simulink model "sampleModel2432_pp_1_2"  (R2018a)
settings: Solver=VariableStepAuto  StartTime=0.0  StopTime=10.0  RelTol=1e-3
undefined symbols (not defined in the file or in its folder): DiscIntNeverNeededParam, sigbuilder_block
libraries: simulink x302
(part 6 of 7)

== system sampleModel2432_pp_1_2/cfblk225/cfblk17 ==
  cfblk1 : Inport
  Action Port : ActionPort
  cfblk{10,15..17} (4 alike) : Delay
  cfblk14 : simulink/Discrete/Transfer Fcn Lead or Lag  PoleZ=0.95  ZeroZ=0.75  ICPrevOutput=0.0  ICPrevInput=0.0  DoSatur=off
      settings: SourceProductName=Simulink  SourceProductBaseCode=SL
  cfblk3 : DiscreteFilter
  cfblk4 : simulink/Continuous/PID Controller (2DOF)  Controller=PID  TimeDomain=Discrete-time  SampleTime=-1  IntegratorMethod=Forward Euler  FilterMethod=Forward Euler  Form=Parallel  UseFilter=on  ControllerParametersSource=internal  P=1  I=1  D=0  N=100  b=1  c=1  InitialConditionSource=internal  InitialConditionForIntegrator=0  InitialConditionForFilter=0  ExternalReset=none  LimitOutput=off  UpperSaturationLimit=inf  LowerSaturationLimit=-inf  LinearizeAsGain=off  AntiWindupMode=none  Kb=1  TrackingMode=off  Kt=1  PParamMin=[]  PParamMax=[]  IParamMin=[]  IParamMax=[]  DParamMin=[]  DParamMax=[]  NParamMin=[]  NParamMax=[]  bParamMin=[]  bParamMax=[]  cParamMin=[]  cParamMax=[]  KbParamMin=[]  KbParamMax=[]  KtParamMin=[]  KtParamMax=[]  POutMin=[]  POutMax=[]  IOutMin=[]  IOutMax=[]  DOutMin=[]  DOutMax=[]  NOutMin=[]  NOutMax=[]  bOutMin=[]  bOutMax=[]  cOutMin=[]  cOutMax=[]  KbOutMin=[]  KbOutMax=[]  KtOutMin=[]  KtOutMax=[]  IntegratorOutMin=[]  IntegratorOutMax=[]  FilterOutMin=[]  FilterOutMax=[]  SumOutMin=[]  SumOutMax=[]  Sum1OutMin=[]  Sum1OutMax=[]  Sum2OutMin=[]  Sum2OutMax=[]  Sum3OutMin=[]  Sum3OutMax=[]  SumI1OutMin=[]  SumI1OutMax=[]  SumI2OutMin=[]  SumI2OutMax=[]  SumI3OutMin=[]  SumI3OutMax=[]  SumDOutMin=[]  SumDOutMax=[]  SaturationOutMin=[]  SaturationOutMax=[]  IntegratorContinuousStateAttributes=''  IntegratorStateMustResolveToSignalObject=off  IntegratorRTWStateStorageClass=Auto  FilterContinuousStateAttributes=''  FilterStateMustResolveToSignalObject=off  FilterRTWStateStorageClass=Auto  DifferentiatorICPrevScaledInput=0  DifferentiatorOutMin=[]  DifferentiatorOutMax=[]  FilterDiffOutCoefMin=[]  FilterDiffOutCoefMax=[]  SumDenOutMin=[]  SumDenOutMax=[]  SumNumOutMin=[]  SumNumOutMax=[]  ReciprocalOutMin=[]  ReciprocalOutMax=[]  DivideOutMin=[]  DivideOutMax=[]  TunerSelectOption=Transfer Function Based (PID Tuner App)
  cfblk6 : DiscreteStateSpace  SampleTime=-1
  cfblk7 : DiscreteTransferFcn
  cfblk8 : Delay  DelayLengthSource=Input port
      settings: InputPortMap=u0,p1
  cyemi_{709..726} (18 alike) : DataTypeConversion  OutDataTypeStr=double
  cfblk2 : Outport
  wires:
  cfblk1/1 -> cyemi_709/1, cyemi_719/1
  cfblk6/1 -> cfblk2/1
  cyemi_709/1 -> cfblk10/1
  cfblk8/1 -> cyemi_710/1
  cyemi_713/1 -> cfblk14/1
  cyemi_714/1 -> cfblk15/1
  cfblk7/1 -> cyemi_714/1
  cyemi_715/1 -> cfblk16/1
  cyemi_716/1 -> cfblk17/1
  cyemi_717/1 -> cfblk3/1
  cfblk4/1 -> cyemi_717/1
  cyemi_718/1 -> cfblk4/1
  cfblk15/1 -> cyemi_718/1
  cyemi_719/1 -> cfblk4/2
  cyemi_721/1 -> cfblk6/1
  cfblk10/1 -> cyemi_721/1
  cyemi_722/1 -> cfblk7/1
  cfblk14/1 -> cyemi_722/1
  cyemi_723/1 -> cfblk8/1
  cfblk3/1 -> cyemi_723/1
  cyemi_724/1 -> cfblk8/2
  cfblk17/1 -> cyemi_724/1
  cfblk16/1 -> cyemi_725/1
  cyemi_725/1 -> cyemi_720/1
  cyemi_711/1 -> cyemi_715/1
  cyemi_712/1 -> cyemi_726/1, cyemi_713/1
  cyemi_710/1 -> cyemi_716/1, cyemi_712/1
  cyemi_720/1 -> cyemi_711/1

== system sampleModel2432_pp_1_2/cfblk227/cfblk13 ==
  cfblk1 : Inport
  cfblk13 : Inport  Port=2
  cfblk14 : Inport  Port=3
  Action Port : ActionPort  ActionType=then
  cfblk10 : Delay  DelayLengthSource=Input port
      settings: InputPortMap=u0,p1
  cfblk11 : simulink/Discrete/Difference  ICPrevInput=0.0  OutMin=[]  OutMax=[]  OutDataTypeStr=Inherit: Inherit via back propagation  OutDataType=fixdt(1, 16)  OutScaling=2^-10  DoSatur=off
  cfblk16 : Delay
  cfblk3 : simulink/Discrete/Difference  ICPrevInput=0.0  OutMin=[]  OutMax=[]  OutDataTypeStr=Inherit: Inherit via back propagation  OutDataType=fixdt(1, 16)  OutScaling=2^-10  DoSatur=off
  cfblk5 : UnitDelay  SampleTime=-1
  cfblk6 : Delay
  cfblk7 : Delay  ShowEnablePort=on
      settings: InputPortMap=u0,e6
  cfblk9 : simulink/Discrete/Transfer Fcn Real Zero  ZeroZ=0.75  ICPrevInput=0.0  DoSatur=off
      settings: SourceProductName=Simulink  SourceProductBaseCode=SL
  cyemi_{761..774} (14 alike) : DataTypeConversion  OutDataTypeStr=double
  cfblk2 : Outport
  cfblk15 : Outport  Port=2
  wires:
  cfblk3/1 -> cfblk2/1
  cfblk13/1 -> cyemi_763/1, cyemi_774/1
  cyemi_761/1 -> cfblk10/1
  cfblk14/1 -> cyemi_761/1
  cyemi_762/1 -> cfblk10/2
  cfblk5/1 -> cyemi_762/1
  cyemi_763/1 -> cfblk11/1
  cfblk11/1 -> cyemi_764/1
  cfblk6/1 -> cyemi_765/1
  cyemi_766/1 -> cfblk16/1
  cyemi_767/1 -> cfblk3/1
  cfblk9/1 -> cyemi_768/1
  cyemi_769/1 -> cfblk5/1
  cyemi_770/1 -> cfblk6/1
  cfblk7/1 -> cyemi_770/1
  cyemi_771/1 -> cfblk7/1
  cfblk10/1 -> cyemi_771/1
  cyemi_772/1 -> cfblk7/2
  cfblk16/1 -> cyemi_772/1
  cfblk1/1 -> cyemi_773/1
  cyemi_774/1 -> cfblk9/1
  cyemi_768/1 -> cyemi_769/1, cfblk15/1
  cyemi_764/1 -> cyemi_766/1
  cyemi_773/1 -> cyemi_767/1

== system sampleModel2432_pp_1_2/cfblk227/cfblk14 ==
  cfblk1 : Inport
  cfblk6 : Inport  Port=2
  Action Port : ActionPort  ActionType=else
  cfblk3 : simulink/Discrete/Tapped Delay  vinit=0.0  samptime=-1  NumDelays=1  DelayOrder=Oldest  includeCurrent=off
  cfblk4 : simulink/Discrete/Difference  ICPrevInput=0.0  OutMin=[]  OutMax=[]  OutDataTypeStr=Inherit: Inherit via back propagation  OutDataType=fixdt(1, 16)  OutScaling=2^-10  DoSatur=off
  cyemi_777 : DataTypeConversion  OutDataTypeStr=double
  cyemi_778 : DataTypeConversion  OutDataTypeStr=double
  cyemi_779 : DataTypeConversion  OutDataTypeStr=double
  cfblk2 : Outport
  cfblk7 : Outport  Port=2
  wires:
  cfblk3/1 -> cfblk2/1
  cfblk4/1 -> cfblk7/1
  cyemi_777/1 -> cfblk3/1
  cfblk6/1 -> cyemi_777/1
  cyemi_778/1 -> cfblk4/1
  cfblk1/1 -> cyemi_779/1
  cyemi_779/1 -> cyemi_778/1

== system sampleModel2432_pp_1_2/cfblk230/cfblk10 ==
  cfblk1 : Inport
  Action Port : ActionPort  ActionType=then
  cfblk10 : UnitDelay  SampleTime=-1
  cfblk13 : Delay
  cfblk14 : Delay
  cfblk3 : simulink/Continuous/PID Controller (2DOF)  Controller=PID  TimeDomain=Discrete-time  SampleTime=-1  IntegratorMethod=Forward Euler  FilterMethod=Forward Euler  Form=Parallel  UseFilter=on  ControllerParametersSource=internal  P=1  I=1  D=0  N=100  b=1  c=1  InitialConditionSource=internal  InitialConditionForIntegrator=0  InitialConditionForFilter=0  ExternalReset=none  LimitOutput=off  UpperSaturationLimit=inf  LowerSaturationLimit=-inf  LinearizeAsGain=off  AntiWindupMode=none  Kb=1  TrackingMode=off  Kt=1  PParamMin=[]  PParamMax=[]  IParamMin=[]  IParamMax=[]  DParamMin=[]  DParamMax=[]  NParamMin=[]  NParamMax=[]  bParamMin=[]  bParamMax=[]  cParamMin=[]  cParamMax=[]  KbParamMin=[]  KbParamMax=[]  KtParamMin=[]  KtParamMax=[]  POutMin=[]  POutMax=[]  IOutMin=[]  IOutMax=[]  DOutMin=[]  DOutMax=[]  NOutMin=[]  NOutMax=[]  bOutMin=[]  bOutMax=[]  cOutMin=[]  cOutMax=[]  KbOutMin=[]  KbOutMax=[]  KtOutMin=[]  KtOutMax=[]  IntegratorOutMin=[]  IntegratorOutMax=[]  FilterOutMin=[]  FilterOutMax=[]  SumOutMin=[]  SumOutMax=[]  Sum1OutMin=[]  Sum1OutMax=[]  Sum2OutMin=[]  Sum2OutMax=[]  Sum3OutMin=[]  Sum3OutMax=[]  SumI1OutMin=[]  SumI1OutMax=[]  SumI2OutMin=[]  SumI2OutMax=[]  SumI3OutMin=[]  SumI3OutMax=[]  SumDOutMin=[]  SumDOutMax=[]  SaturationOutMin=[]  SaturationOutMax=[]  IntegratorContinuousStateAttributes=''  IntegratorStateMustResolveToSignalObject=off  IntegratorRTWStateStorageClass=Auto  FilterContinuousStateAttributes=''  FilterStateMustResolveToSignalObject=off  FilterRTWStateStorageClass=Auto  DifferentiatorICPrevScaledInput=0  DifferentiatorOutMin=[]  DifferentiatorOutMax=[]  FilterDiffOutCoefMin=[]  FilterDiffOutCoefMax=[]  SumDenOutMin=[]  SumDenOutMax=[]  SumNumOutMin=[]  SumNumOutMax=[]  ReciprocalOutMin=[]  ReciprocalOutMax=[]  DivideOutMin=[]  DivideOutMax=[]  TunerSelectOption=Transfer Function Based (PID Tuner App)
  cfblk5 : DiscreteFir
  cfblk6 : UnitDelay  SampleTime=-1
  cfblk8 : simulink/Continuous/PID Controller  Controller=PID  TimeDomain=Discrete-time  SampleTime=-1  IntegratorMethod=Forward Euler  FilterMethod=Forward Euler  Form=Parallel  UseFilter=on  ControllerParametersSource=internal  P=1  I=1  D=0  N=100  InitialConditionSource=internal  InitialConditionForIntegrator=0  InitialConditionForFilter=0  ExternalReset=none  LimitOutput=off  UpperSaturationLimit=inf  LowerSaturationLimit=-inf  LinearizeAsGain=off  AntiWindupMode=none  Kb=1  TrackingMode=off  Kt=1  PParamMin=[]  PParamMax=[]  IParamMin=[]  IParamMax=[]  DParamMin=[]  DParamMax=[]  NParamMin=[]  NParamMax=[]  KbParamMin=[]  KbParamMax=[]  KtParamMin=[]  KtParamMax=[]  POutMin=[]  POutMax=[]  IOutMin=[]  IOutMax=[]  DOutMin=[]  DOutMax=[]  NOutMin=[]  NOutMax=[]  KbOutMin=[]  KbOutMax=[]  KtOutMin=[]  KtOutMax=[]  IntegratorOutMin=[]  IntegratorOutMax=[]  FilterOutMin=[]  FilterOutMax=[]  SumOutMin=[]  SumOutMax=[]  SumI1OutMin=[]  SumI1OutMax=[]  SumI2OutMin=[]  SumI2OutMax=[]  SumI3OutMin=[]  SumI3OutMax=[]  SumDOutMin=[]  SumDOutMax=[]  SaturationOutMin=[]  SaturationOutMax=[]  IntegratorContinuousStateAttributes=''  IntegratorStateMustResolveToSignalObject=off  IntegratorRTWStateStorageClass=Auto  FilterContinuousStateAttributes=''  FilterStateMustResolveToSignalObject=off  FilterRTWStateStorageClass=Auto  DifferentiatorICPrevScaledInput=0  DifferentiatorOutMin=[]  DifferentiatorOutMax=[]  FilterDiffOutCoefMin=[]  FilterDiffOutCoefMax=[]  SumDenOutMin=[]  SumDenOutMax=[]  SumNumOutMin=[]  SumNumOutMax=[]  ReciprocalOutMin=[]  ReciprocalOutMax=[]  DivideOutMin=[]  DivideOutMax=[]  TunerSelectOption=Transfer Function Based (PID Tuner App)
  cyemi_{816..826} (11 alike) : DataTypeConversion  OutDataTypeStr=double
  cfblk2 : Outport
  cfblk11 : Outport  Port=2
  cfblk12 : Outport  Port=3
  wires:
  cfblk10/1 -> cfblk12/1, cyemi_821/1
  cfblk6/1 -> cyemi_817/1, cyemi_822/1
  cfblk8/1 -> cfblk2/1
  cfblk5/1 -> cfblk11/1
  cyemi_816/1 -> cfblk10/1
  cfblk3/1 -> cyemi_816/1
  cyemi_817/1 -> cfblk13/1
  cyemi_818/1 -> cfblk14/1
  cyemi_819/1 -> cfblk3/1
  cfblk14/1 -> cyemi_819/1
  cyemi_820/1 -> cfblk3/2
  cfblk13/1 -> cyemi_820/1
  cyemi_822/1 -> cfblk5/1
  cyemi_823/1 -> cfblk6/1
  cyemi_825/1 -> cfblk8/1
  cfblk1/1 -> cyemi_825/1
  cyemi_826/1 -> cyemi_818/1
  cyemi_821/1 -> cyemi_824/1
  cyemi_824/1 -> cyemi_826/1, cyemi_823/1

== system sampleModel2432_pp_1_2/cfblk230/cfblk11 ==
  cfblk1 : Inport
  Action Port : ActionPort  ActionType=else
  cfblk12 : Delay
  cfblk3 : simulink/Discrete/Transfer Fcn Lead or Lag  PoleZ=0.95  ZeroZ=0.75  ICPrevOutput=0.0  ICPrevInput=0.0  DoSatur=off
      settings: SourceProductName=Simulink  SourceProductBaseCode=SL
  cfblk4 : Delay  ShowEnablePort=on
      settings: InputPortMap=u0,e6
  cfblk5 : simulink/Discrete/Tapped Delay  vinit=0.0  samptime=-1  NumDelays=1  DelayOrder=Oldest  includeCurrent=off
  cfblk6 : Delay  ShowEnablePort=on
      settings: InputPortMap=u0,e6
  cfblk7 : simulink/Discrete/Transfer Fcn Real Zero  ZeroZ=0.75  ICPrevInput=0.0  DoSatur=off
      settings: SourceProductName=Simulink  SourceProductBaseCode=SL
  cfblk8 : simulink/Discrete/Transfer Fcn First Order  PoleZ=0.95  ICPrevOutput=0.0  DoSatur=off
      settings: SourceProductName=Simulink
  cfblk9 : DiscreteStateSpace  SampleTime=-1
  cyemi_{828..837} (10 alike) : DataTypeConversion  OutDataTypeStr=double
  cfblk2 : Outport
  cfblk10 : Outport  Port=2
  cfblk11 : Outport  Port=3
  wires:
  cfblk1/1 -> cyemi_830/1, cyemi_837/1
  cfblk9/1 -> cyemi_834/1, cyemi_835/1
  cfblk8/1 -> cfblk2/1
  cfblk3/1 -> cyemi_828/1, cyemi_833/1
  cfblk7/1 -> cfblk11/1
  cfblk5/1 -> cfblk10/1, cyemi_829/1
  cyemi_828/1 -> cfblk12/1
  cyemi_829/1 -> cfblk3/1
  cyemi_830/1 -> cfblk4/1
  cyemi_831/1 -> cfblk4/2
  cfblk12/1 -> cyemi_831/1
  cyemi_832/1 -> cfblk5/1
  cfblk4/1 -> cyemi_832/1
  cyemi_833/1 -> cfblk6/1
  cyemi_834/1 -> cfblk6/2
  cyemi_835/1 -> cfblk7/1
  cyemi_836/1 -> cfblk8/1
  cfblk6/1 -> cyemi_836/1
  cyemi_837/1 -> cfblk9/1

== system sampleModel2432_pp_1_2/cfblk231/cfblk14 ==
  cfblk1 : Inport
  cfblk6 : Inport  Port=2
  cfblk7 : Inport  Port=3
  cfblk8 : Inport  Port=4
  cfblk9 : Inport  Port=5
  Action Port : ActionPort  ActionType=then
  cfblk3 : simulink/Discrete/Difference  ICPrevInput=0.0  OutMin=[]  OutMax=[]  OutDataTypeStr=Inherit: Inherit via back propagation  OutDataType=fixdt(1, 16)  OutScaling=2^-10  DoSatur=off
  cyemi_856 : DataTypeConversion  OutDataTypeStr=double
  cyemi_857 : DataTypeConversion  OutDataTypeStr=double
  cyemi_858 : DataTypeConversion  OutDataTypeStr=double
  cfblk2 : Outport
  cfblk10 : Outport  Port=2
  cfblk11 : Outport  Port=3
  wires:
  cfblk6/1 -> cfblk10/1
  cfblk8/1 -> cfblk11/1
  cfblk3/1 -> cfblk2/1
  cyemi_856/1 -> cfblk3/1
  cfblk9/1 -> cyemi_857/1
  cfblk1/1 -> cyemi_858/1
  cyemi_857/1 -> cyemi_856/1

== system sampleModel2432_pp_1_2/cfblk231/cfblk15 ==
  cfblk1 : Inport
  Action Port : ActionPort  ActionType=else
  cfblk3 : Delay
  cfblk4 : simulink/Continuous/PID Controller (2DOF)  Controller=PID  TimeDomain=Discrete-time  SampleTime=-1  IntegratorMethod=Forward Euler  FilterMethod=Forward Euler  Form=Parallel  UseFilter=on  ControllerParametersSource=internal  P=1  I=1  D=0  N=100  b=1  c=1  InitialConditionSource=internal  InitialConditionForIntegrator=0  InitialConditionForFilter=0  ExternalReset=none  LimitOutput=off  UpperSaturationLimit=inf  LowerSaturationLimit=-inf  LinearizeAsGain=off  AntiWindupMode=none  Kb=1  TrackingMode=off  Kt=1  PParamMin=[]  PParamMax=[]  IParamMin=[]  IParamMax=[]  DParamMin=[]  DParamMax=[]  NParamMin=[]  NParamMax=[]  bParamMin=[]  bParamMax=[]  cParamMin=[]  cParamMax=[]  KbParamMin=[]  KbParamMax=[]  KtParamMin=[]  KtParamMax=[]  POutMin=[]  POutMax=[]  IOutMin=[]  IOutMax=[]  DOutMin=[]  DOutMax=[]  NOutMin=[]  NOutMax=[]  bOutMin=[]  bOutMax=[]  cOutMin=[]  cOutMax=[]  KbOutMin=[]  KbOutMax=[]  KtOutMin=[]  KtOutMax=[]  IntegratorOutMin=[]  IntegratorOutMax=[]  FilterOutMin=[]  FilterOutMax=[]  SumOutMin=[]  SumOutMax=[]  Sum1OutMin=[]  Sum1OutMax=[]  Sum2OutMin=[]  Sum2OutMax=[]  Sum3OutMin=[]  Sum3OutMax=[]  SumI1OutMin=[]  SumI1OutMax=[]  SumI2OutMin=[]  SumI2OutMax=[]  SumI3OutMin=[]  SumI3OutMax=[]  SumDOutMin=[]  SumDOutMax=[]  SaturationOutMin=[]  SaturationOutMax=[]  IntegratorContinuousStateAttributes=''  IntegratorStateMustResolveToSignalObject=off  IntegratorRTWStateStorageClass=Auto  FilterContinuousStateAttributes=''  FilterStateMustResolveToSignalObject=off  FilterRTWStateStorageClass=Auto  DifferentiatorICPrevScaledInput=0  DifferentiatorOutMin=[]  DifferentiatorOutMax=[]  FilterDiffOutCoefMin=[]  FilterDiffOutCoefMax=[]  SumDenOutMin=[]  SumDenOutMax=[]  SumNumOutMin=[]  SumNumOutMax=[]  ReciprocalOutMin=[]  ReciprocalOutMax=[]  DivideOutMin=[]  DivideOutMax=[]  TunerSelectOption=Transfer Function Based (PID Tuner App)
  cfblk5 : Delay  ShowEnablePort=on
      settings: InputPortMap=u0,e6
  cfblk9 : Delay
  cyemi_{860..865} (6 alike) : DataTypeConversion  OutDataTypeStr=double
  cfblk2 : Outport
  cfblk6 : Outport  Port=2
  cfblk7 : Outport  Port=3
  cfblk8 : Outport  Port=4
  wires:
  cfblk1/1 -> cfblk6/1, cyemi_864/1
  cfblk3/1 -> cfblk2/1, cfblk8/1, cfblk7/1, cyemi_861/1
  cfblk5/1 -> cyemi_860/1, cyemi_862/1
  cyemi_860/1 -> cfblk3/1
  cyemi_861/1 -> cfblk4/1
  cyemi_862/1 -> cfblk4/2
  cyemi_863/1 -> cfblk5/1
  cfblk9/1 -> cyemi_863/1
  cyemi_864/1 -> cfblk5/2
  cyemi_865/1 -> cfblk9/1
  cfblk4/1 -> cyemi_865/1

== system sampleModel2432_pp_1_2/cfblk234/cfblk8 ==
  cfblk1 : Inport
  Action Port : ActionPort  ActionType=then
  cfblk3 : simulink/Discrete/Transfer Fcn Real Zero  ZeroZ=0.75  ICPrevInput=0.0  DoSatur=off
      settings: SourceProductName=Simulink  SourceProductBaseCode=SL
  cfblk4 : Delay
  cfblk5 : UnitDelay  SampleTime=-1
  cfblk8 : Delay
  cfblk9 : Delay
  cyemi_{907..913} (7 alike) : DataTypeConversion  OutDataTypeStr=double
  cfblk2 : Outport
  wires:
  cfblk1/1 -> cfblk2/1
  cyemi_907/1 -> cfblk3/1
  cfblk8/1 -> cyemi_907/1
  cyemi_908/1 -> cfblk4/1
  cfblk3/1 -> cyemi_908/1
  cyemi_909/1 -> cfblk5/1
  cfblk4/1 -> cyemi_909/1
  cfblk9/1 -> cyemi_910/1
  cyemi_912/1 -> cfblk8/1
  cfblk5/1 -> cyemi_912/1
  cyemi_913/1 -> cfblk9/1
  cyemi_910/1 -> cyemi_911/1
  cyemi_911/1 -> cyemi_913/1

== system sampleModel2432_pp_1_2/cfblk234/cfblk9 ==
  cfblk1 : Inport
  Action Port : ActionPort  ActionType=else
  cfblk11 : Delay
  cfblk12 : Delay
  cfblk3 : Delay  DelayLengthSource=Input port
      settings: InputPortMap=u0,p1
  cfblk4 : simulink/Discrete/Tapped Delay  vinit=0.0  samptime=-1  NumDelays=1  DelayOrder=Oldest  includeCurrent=off
  cfblk5 : DiscreteIntegrator  SampleTime=-1  ICPrevOutput=DiscIntNeverNeededParam  ICPrevScaledInput=DiscIntNeverNeededParam
  cfblk6 : DiscreteFir
  cfblk7 : DiscreteFir
  cfblk8 : DiscreteTransferFcn
  cfblk9 : Delay
  cyemi_{915..924} (10 alike) : DataTypeConversion  OutDataTypeStr=double
  cfblk2 : Outport
  cfblk10 : Outport  Port=2
  wires:
  cfblk5/1 -> cfblk2/1
  cfblk4/1 -> cfblk10/1
  cfblk1/1 -> cyemi_918/1, cyemi_919/1
  cfblk3/1 -> cyemi_920/1, cyemi_921/1
  cyemi_915/1 -> cfblk11/1
  cfblk7/1 -> cyemi_915/1
  cyemi_916/1 -> cfblk12/1
  cfblk9/1 -> cyemi_916/1
  cyemi_917/1 -> cfblk3/1
  cfblk11/1 -> cyemi_917/1
  cyemi_918/1 -> cfblk3/2
  cyemi_919/1 -> cfblk4/1
  cyemi_920/1 -> cfblk5/1
  cyemi_921/1 -> cfblk6/1
  cyemi_922/1 -> cfblk7/1
  cfblk6/1 -> cyemi_922/1
  cyemi_923/1 -> cfblk8/1
  cfblk12/1 -> cyemi_923/1
  cyemi_924/1 -> cfblk9/1
  cfblk8/1 -> cyemi_924/1

== system sampleModel2432_pp_1_2/cfblk237/cfblk16 ==
  cfblk1 : Inport
  cfblk16 : Inport  Port=2
  Action Port : ActionPort
  cfblk11 : UnitDelay  SampleTime=-1
  cfblk12 : simulink/Discrete/Transfer Fcn Lead or Lag  PoleZ=0.95  ZeroZ=0.75  ICPrevOutput=0.0  ICPrevInput=0.0  DoSatur=off
      settings: SourceProductName=Simulink  SourceProductBaseCode=SL
  cfblk13 : DiscreteTransferFcn
  cfblk14 : DiscreteFilter
  cfblk15 : Delay  ShowEnablePort=on
      settings: InputPortMap=u0,e6
  cfblk17 : Delay
  cfblk18 : Delay
  cfblk6 : simulink/Discrete/Transfer Fcn Lead or Lag  PoleZ=0.95  ZeroZ=0.75  ICPrevOutput=0.0  ICPrevInput=0.0  DoSatur=off
      settings: SourceProductName=Simulink  SourceProductBaseCode=SL
  cfblk7 : DiscreteZeroPole  Poles=[0 0.5]  Gain=1  SampleTime=-1
  cfblk9 : simulink/Discrete/Transfer Fcn Lead or Lag  PoleZ=0.95  ZeroZ=0.75  ICPrevOutput=0.0  ICPrevInput=0.0  DoSatur=off
      settings: SourceProductName=Simulink  SourceProductBaseCode=SL
  cyemi_{956..971} (16 alike) : DataTypeConversion  OutDataTypeStr=double
  cfblk2 : Outport
  wires:
  cfblk13/1 -> cfblk2/1
  cyemi_957/1 -> cfblk11/1
  cfblk15/1 -> cyemi_957/1
  cyemi_958/1 -> cfblk12/1
  cfblk6/1 -> cyemi_958/1
  cyemi_959/1 -> cfblk13/1
  cfblk16/1 -> cyemi_959/1
  cyemi_960/1 -> cfblk14/1
  cfblk1/1 -> cyemi_960/1
  cyemi_961/1 -> cfblk15/1
  cyemi_962/1 -> cfblk15/2
  cfblk17/1 -> cyemi_962/1
  cyemi_963/1 -> cfblk17/1
  cfblk11/1 -> cyemi_963/1
  cyemi_964/1 -> cfblk18/1
  cfblk9/1 -> cyemi_964/1
  cfblk7/1 -> cyemi_965/1
  cfblk14/1 -> cyemi_966/1
  cfblk18/1 -> cyemi_967/1
  cyemi_968/1 -> cfblk6/1
  cyemi_969/1 -> cfblk7/1
  cyemi_971/1 -> cfblk9/1
  cfblk12/1 -> cyemi_971/1
  cyemi_970/1 -> cyemi_968/1
  cyemi_966/1 -> cyemi_969/1
  cyemi_967/1 -> cyemi_956/1
  cyemi_956/1 -> cyemi_970/1
  cyemi_965/1 -> cyemi_961/1

== system sampleModel2432_pp_1_2/cfblk237/cfblk17 ==
  cfblk1 : Inport
  cfblk10 : Inport  Port=2
  cfblk11 : Inport  Port=3
  cfblk12 : Inport  Port=4
  Action Port : ActionPort
  cfblk13 : Delay
  cfblk3 : DiscreteFilter
  cfblk4 : simulink/Discrete/Difference  ICPrevInput=0.0  OutMin=[]  OutMax=[]  OutDataTypeStr=Inherit: Inherit via back propagation  OutDataType=fixdt(1, 16)  OutScaling=2^-10  DoSatur=off
  cfblk5 : Delay  ShowEnablePort=on
      settings: InputPortMap=u0,e6
  cfblk6 : simulink/Discrete/Tapped Delay  vinit=0.0  samptime=-1  NumDelays=1  DelayOrder=Oldest  includeCurrent=off
  cfblk7 : simulink/Discrete/Transfer Fcn Lead or Lag  PoleZ=0.95  ZeroZ=0.75  ICPrevOutput=0.0  ICPrevInput=0.0  DoSatur=off
      settings: SourceProductName=Simulink  SourceProductBaseCode=SL
  cfblk8 : simulink/Continuous/PID Controller (2DOF)  Controller=PID  TimeDomain=Discrete-time  SampleTime=-1  IntegratorMethod=Forward Euler  FilterMethod=Forward Euler  Form=Parallel  UseFilter=on  ControllerParametersSource=internal  P=1  I=1  D=0  N=100  b=1  c=1  InitialConditionSource=internal  InitialConditionForIntegrator=0  InitialConditionForFilter=0  ExternalReset=none  LimitOutput=off  UpperSaturationLimit=inf  LowerSaturationLimit=-inf  LinearizeAsGain=off  AntiWindupMode=none  Kb=1  TrackingMode=off  Kt=1  PParamMin=[]  PParamMax=[]  IParamMin=[]  IParamMax=[]  DParamMin=[]  DParamMax=[]  NParamMin=[]  NParamMax=[]  bParamMin=[]  bParamMax=[]  cParamMin=[]  cParamMax=[]  KbParamMin=[]  KbParamMax=[]  KtParamMin=[]  KtParamMax=[]  POutMin=[]  POutMax=[]  IOutMin=[]  IOutMax=[]  DOutMin=[]  DOutMax=[]  NOutMin=[]  NOutMax=[]  bOutMin=[]  bOutMax=[]  cOutMin=[]  cOutMax=[]  KbOutMin=[]  KbOutMax=[]  KtOutMin=[]  KtOutMax=[]  IntegratorOutMin=[]  IntegratorOutMax=[]  FilterOutMin=[]  FilterOutMax=[]  SumOutMin=[]  SumOutMax=[]  Sum1OutMin=[]  Sum1OutMax=[]  Sum2OutMin=[]  Sum2OutMax=[]  Sum3OutMin=[]  Sum3OutMax=[]  SumI1OutMin=[]  SumI1OutMax=[]  SumI2OutMin=[]  SumI2OutMax=[]  SumI3OutMin=[]  SumI3OutMax=[]  SumDOutMin=[]  SumDOutMax=[]  SaturationOutMin=[]  SaturationOutMax=[]  IntegratorContinuousStateAttributes=''  IntegratorStateMustResolveToSignalObject=off  IntegratorRTWStateStorageClass=Auto  FilterContinuousStateAttributes=''  FilterStateMustResolveToSignalObject=off  FilterRTWStateStorageClass=Auto  DifferentiatorICPrevScaledInput=0  DifferentiatorOutMin=[]  DifferentiatorOutMax=[]  FilterDiffOutCoefMin=[]  FilterDiffOutCoefMax=[]  SumDenOutMin=[]  SumDenOutMax=[]  SumNumOutMin=[]  SumNumOutMax=[]  ReciprocalOutMin=[]  ReciprocalOutMax=[]  DivideOutMin=[]  DivideOutMax=[]  TunerSelectOption=Transfer Function Based (PID Tuner App)
  cfblk9 : DiscreteTransferFcn
  cyemi_{976..985} (10 alike) : DataTypeConversion  OutDataTypeStr=double
  cfblk2 : Outport
  wires:
  cfblk10/1 -> cfblk2/1
  cyemi_976/1 -> cfblk13/1
  cfblk9/1 -> cyemi_976/1
  cyemi_977/1 -> cfblk3/1
  cfblk1/1 -> cyemi_977/1
  cyemi_978/1 -> cfblk4/1
  cfblk7/1 -> cyemi_978/1
  cyemi_979/1 -> cfblk5/1
  cfblk13/1 -> cyemi_979/1
  cyemi_980/1 -> cfblk5/2
  cfblk4/1 -> cyemi_980/1
  cyemi_981/1 -> cfblk6/1
  cfblk12/1 -> cyemi_981/1
  cyemi_982/1 -> cfblk7/1
  cfblk8/1 -> cyemi_982/1
  cyemi_983/1 -> cfblk8/1
  cfblk3/1 -> cyemi_983/1
  cyemi_984/1 -> cfblk8/2
  cfblk6/1 -> cyemi_984/1
  cyemi_985/1 -> cfblk9/1
  cfblk5/1 -> cyemi_985/1

== system sampleModel2432_pp_1_2/cfblk239/cfblk12 ==
  cfblk1 : Inport
  cfblk12 : Inport  Port=2
  Action Port : ActionPort  ActionType=then
  cfblk10 : Delay  DelayLengthSource=Input port
      settings: InputPortMap=u0,p1
  cfblk11 : simulink/Discrete/Tapped Delay  vinit=0.0  samptime=-1  NumDelays=1  DelayOrder=Oldest  includeCurrent=off
  cfblk3 : DiscreteFilter
  cfblk4 : Delay  ShowEnablePort=on
      settings: InputPortMap=u0,e6
  cfblk5 : DiscreteStateSpace  SampleTime=-1
  cfblk6 : simulink/Discrete/Transfer Fcn Lead or Lag  PoleZ=0.95  ZeroZ=0.75  ICPrevOutput=0.0  ICPrevInput=0.0  DoSatur=off
      settings: SourceProductName=Simulink  SourceProductBaseCode=SL
  cfblk7 : DiscreteTransferFcn
  cfblk8 : DiscreteStateSpace  SampleTime=-1
  cfblk9 : DiscreteZeroPole  Poles=[0 0.5]  Gain=1  SampleTime=-1
  cyemi_{1021..1031} (11 alike) : DataTypeConversion  OutDataTypeStr=double
  cfblk2 : Outport
  cfblk13 : Outport  Port=2
  cfblk14 : Outport  Port=3
  wires:
  cfblk9/1 -> cyemi_1022/1, cyemi_1023/1
  cfblk3/1 -> cfblk14/1
  cfblk11/1 -> cyemi_1025/1, cyemi_1029/1
  cfblk1/1 -> cyemi_1021/1, cyemi_1031/1
  cfblk8/1 -> cfblk13/1
  cfblk6/1 -> cfblk2/1
  cyemi_1021/1 -> cfblk10/1
  cyemi_1022/1 -> cfblk10/2
  cyemi_1023/1 -> cfblk11/1
  cyemi_1024/1 -> cfblk3/1
  cfblk12/1 -> cyemi_1024/1
  cyemi_1025/1 -> cfblk4/1
  cyemi_1026/1 -> cfblk4/2
  cfblk7/1 -> cyemi_1026/1
  cyemi_1027/1 -> cfblk5/1
  cfblk4/1 -> cyemi_1027/1
  cyemi_1028/1 -> cfblk6/1
  cfblk10/1 -> cyemi_1028/1
  cyemi_1029/1 -> cfblk7/1
  cyemi_1030/1 -> cfblk8/1
  cfblk5/1 -> cyemi_1030/1
  cyemi_1031/1 -> cfblk9/1

== system sampleModel2432_pp_1_2/cfblk239/cfblk13 ==
  cfblk1 : Inport
  cfblk11 : Inport  Port=2
  cfblk12 : Inport  Port=3
  cfblk13 : Inport  Port=4
  Action Port : ActionPort  ActionType=else
  cfblk10 : simulink/Continuous/PID Controller  Controller=PID  TimeDomain=Discrete-time  SampleTime=-1  IntegratorMethod=Forward Euler  FilterMethod=Forward Euler  Form=Parallel  UseFilter=on  ControllerParametersSource=internal  P=1  I=1  D=0  N=100  InitialConditionSource=internal  InitialConditionForIntegrator=0  InitialConditionForFilter=0  ExternalReset=none  LimitOutput=off  UpperSaturationLimit=inf  LowerSaturationLimit=-inf  LinearizeAsGain=off  AntiWindupMode=none  Kb=1  TrackingMode=off  Kt=1  PParamMin=[]  PParamMax=[]  IParamMin=[]  IParamMax=[]  DParamMin=[]  DParamMax=[]  NParamMin=[]  NParamMax=[]  KbParamMin=[]  KbParamMax=[]  KtParamMin=[]  KtParamMax=[]  POutMin=[]  POutMax=[]  IOutMin=[]  IOutMax=[]  DOutMin=[]  DOutMax=[]  NOutMin=[]  NOutMax=[]  KbOutMin=[]  KbOutMax=[]  KtOutMin=[]  KtOutMax=[]  IntegratorOutMin=[]  IntegratorOutMax=[]  FilterOutMin=[]  FilterOutMax=[]  SumOutMin=[]  SumOutMax=[]  SumI1OutMin=[]  SumI1OutMax=[]  SumI2OutMin=[]  SumI2OutMax=[]  SumI3OutMin=[]  SumI3OutMax=[]  SumDOutMin=[]  SumDOutMax=[]  SaturationOutMin=[]  SaturationOutMax=[]  IntegratorContinuousStateAttributes=''  IntegratorStateMustResolveToSignalObject=off  IntegratorRTWStateStorageClass=Auto  FilterContinuousStateAttributes=''  FilterStateMustResolveToSignalObject=off  FilterRTWStateStorageClass=Auto  DifferentiatorICPrevScaledInput=0  DifferentiatorOutMin=[]  DifferentiatorOutMax=[]  FilterDiffOutCoefMin=[]  FilterDiffOutCoefMax=[]  SumDenOutMin=[]  SumDenOutMax=[]  SumNumOutMin=[]  SumNumOutMax=[]  ReciprocalOutMin=[]  ReciprocalOutMax=[]  DivideOutMin=[]  DivideOutMax=[]  TunerSelectOption=Transfer Function Based (PID Tuner App)
  cfblk3 : DiscreteFilter
  cfblk4 : simulink/Discrete/Transfer Fcn First Order  PoleZ=0.95  ICPrevOutput=0.0  DoSatur=off
      settings: SourceProductName=Simulink
  cfblk5 : simulink/Continuous/PID Controller  Controller=PID  TimeDomain=Discrete-time  SampleTime=-1  IntegratorMethod=Forward Euler  FilterMethod=Forward Euler  Form=Parallel  UseFilter=on  ControllerParametersSource=internal  P=1  I=1  D=0  N=100  InitialConditionSource=internal  InitialConditionForIntegrator=0  InitialConditionForFilter=0  ExternalReset=none  LimitOutput=off  UpperSaturationLimit=inf  LowerSaturationLimit=-inf  LinearizeAsGain=off  AntiWindupMode=none  Kb=1  TrackingMode=off  Kt=1  PParamMin=[]  PParamMax=[]  IParamMin=[]  IParamMax=[]  DParamMin=[]  DParamMax=[]  NParamMin=[]  NParamMax=[]  KbParamMin=[]  KbParamMax=[]  KtParamMin=[]  KtParamMax=[]  POutMin=[]  POutMax=[]  IOutMin=[]  IOutMax=[]  DOutMin=[]  DOutMax=[]  NOutMin=[]  NOutMax=[]  KbOutMin=[]  KbOutMax=[]  KtOutMin=[]  KtOutMax=[]  IntegratorOutMin=[]  IntegratorOutMax=[]  FilterOutMin=[]  FilterOutMax=[]  SumOutMin=[]  SumOutMax=[]  SumI1OutMin=[]  SumI1OutMax=[]  SumI2OutMin=[]  SumI2OutMax=[]  SumI3OutMin=[]  SumI3OutMax=[]  SumDOutMin=[]  SumDOutMax=[]  SaturationOutMin=[]  SaturationOutMax=[]  IntegratorContinuousStateAttributes=''  IntegratorStateMustResolveToSignalObject=off  IntegratorRTWStateStorageClass=Auto  FilterContinuousStateAttributes=''  FilterStateMustResolveToSignalObject=off  FilterRTWStateStorageClass=Auto  DifferentiatorICPrevScaledInput=0  DifferentiatorOutMin=[]  DifferentiatorOutMax=[]  FilterDiffOutCoefMin=[]  FilterDiffOutCoefMax=[]  SumDenOutMin=[]  SumDenOutMax=[]  SumNumOutMin=[]  SumNumOutMax=[]  ReciprocalOutMin=[]  ReciprocalOutMax=[]  DivideOutMin=[]  DivideOutMax=[]  TunerSelectOption=Transfer Function Based (PID Tuner App)
  cfblk6 : DiscreteTransferFcn
  cfblk7 : simulink/Discrete/Transfer Fcn First Order  PoleZ=0.95  ICPrevOutput=0.0  DoSatur=off
      settings: SourceProductName=Simulink
  cfblk8 : simulink/Continuous/PID Controller (2DOF)  Controller=PID  TimeDomain=Discrete-time  SampleTime=-1  IntegratorMethod=Forward Euler  FilterMethod=Forward Euler  Form=Parallel  UseFilter=on  ControllerParametersSource=internal  P=1  I=1  D=0  N=100  b=1  c=1  InitialConditionSource=internal  InitialConditionForIntegrator=0  InitialConditionForFilter=0  ExternalReset=none  LimitOutput=off  UpperSaturationLimit=inf  LowerSaturationLimit=-inf  LinearizeAsGain=off  AntiWindupMode=none  Kb=1  TrackingMode=off  Kt=1  PParamMin=[]  PParamMax=[]  IParamMin=[]  IParamMax=[]  DParamMin=[]  DParamMax=[]  NParamMin=[]  NParamMax=[]  bParamMin=[]  bParamMax=[]  cParamMin=[]  cParamMax=[]  KbParamMin=[]  KbParamMax=[]  KtParamMin=[]  KtParamMax=[]  POutMin=[]  POutMax=[]  IOutMin=[]  IOutMax=[]  DOutMin=[]  DOutMax=[]  NOutMin=[]  NOutMax=[]  bOutMin=[]  bOutMax=[]  cOutMin=[]  cOutMax=[]  KbOutMin=[]  KbOutMax=[]  KtOutMin=[]  KtOutMax=[]  IntegratorOutMin=[]  IntegratorOutMax=[]  FilterOutMin=[]  FilterOutMax=[]  SumOutMin=[]  SumOutMax=[]  Sum1OutMin=[]  Sum1OutMax=[]  Sum2OutMin=[]  Sum2OutMax=[]  Sum3OutMin=[]  Sum3OutMax=[]  SumI1OutMin=[]  SumI1OutMax=[]  SumI2OutMin=[]  SumI2OutMax=[]  SumI3OutMin=[]  SumI3OutMax=[]  SumDOutMin=[]  SumDOutMax=[]  SaturationOutMin=[]  SaturationOutMax=[]  IntegratorContinuousStateAttributes=''  IntegratorStateMustResolveToSignalObject=off  IntegratorRTWStateStorageClass=Auto  FilterContinuousStateAttributes=''  FilterStateMustResolveToSignalObject=off  FilterRTWStateStorageClass=Auto  DifferentiatorICPrevScaledInput=0  DifferentiatorOutMin=[]  DifferentiatorOutMax=[]  FilterDiffOutCoefMin=[]  FilterDiffOutCoefMax=[]  SumDenOutMin=[]  SumDenOutMax=[]  SumNumOutMin=[]  SumNumOutMax=[]  ReciprocalOutMin=[]  ReciprocalOutMax=[]  DivideOutMin=[]  DivideOutMax=[]  TunerSelectOption=Transfer Function Based (PID Tuner App)
  cfblk9 : Delay
  cyemi_{1036..1044} (9 alike) : DataTypeConversion  OutDataTypeStr=double
  cfblk2 : Outport
  cfblk14 : Outport  Port=2
  cfblk15 : Outport  Port=3
  cfblk16 : Outport  Port=4
  wires:
  cfblk1/1 -> cfblk16/1
  cfblk11/1 -> cfblk2/1, cfblk15/1
  cfblk8/1 -> cfblk14/1
  cyemi_1036/1 -> cfblk10/1
  cfblk5/1 -> cyemi_1036/1
  cyemi_1037/1 -> cfblk3/1
  cfblk7/1 -> cyemi_1037/1
  cyemi_1038/1 -> cfblk4/1
  cfblk10/1 -> cyemi_1038/1
  cyemi_1039/1 -> cfblk5/1
  cfblk6/1 -> cyemi_1039/1
  cyemi_1040/1 -> cfblk6/1
  cfblk9/1 -> cyemi_1040/1
  cyemi_1041/1 -> cfblk7/1
  cfblk4/1 -> cyemi_1041/1
  cyemi_1042/1 -> cfblk8/1
  cfblk3/1 -> cyemi_1042/1
  cyemi_1043/1 -> cfblk8/2
  cfblk12/1 -> cyemi_1043/1
  cyemi_1044/1 -> cfblk9/1
  cfblk13/1 -> cyemi_1044/1

== system sampleModel2432_pp_1_2/cfblk239/cfblk14 ==
  cfblk1 : Inport
  cfblk12 : Inport  Port=2
  cfblk13 : Inport  Port=3
  Action Port : ActionPort  ActionType=then
  cfblk10 : DiscreteZeroPole  Poles=[0 0.5]  Gain=1  SampleTime=-1
  cfblk11 : simulink/Discrete/Transfer Fcn Lead or Lag  PoleZ=0.95  ZeroZ=0.75  ICPrevOutput=0.0  ICPrevInput=0.0  DoSatur=off
      settings: SourceProductName=Simulink  SourceProductBaseCode=SL
  cfblk4 : simulink/Discrete/Difference  ICPrevInput=0.0  OutMin=[]  OutMax=[]  OutDataTypeStr=Inherit: Inherit via back propagation  OutDataType=fixdt(1, 16)  OutScaling=2^-10  DoSatur=off
  cfblk8 : DiscreteFir
  cfblk9 : UnitDelay  SampleTime=-1
  cyemi_{1048..1056} (9 alike) : DataTypeConversion  OutDataTypeStr=double
  cfblk2 : Outport
  wires:
  cfblk11/1 -> cfblk2/1
  cyemi_1048/1 -> cfblk10/1
  cyemi_1049/1 -> cfblk11/1
  cfblk4/1 -> cyemi_1049/1
  cfblk8/1 -> cyemi_1050/1
  cyemi_1051/1 -> cfblk4/1
  cfblk1/1 -> cyemi_1051/1
  cfblk9/1 -> cyemi_1052/1
  cfblk13/1 -> cyemi_1053/1
  cyemi_1055/1 -> cfblk8/1
  cfblk12/1 -> cyemi_1055/1
  cyemi_1056/1 -> cfblk9/1
  cfblk10/1 -> cyemi_1056/1
  cyemi_1050/1 -> cyemi_1054/1
  cyemi_1053/1 -> cyemi_1048/1

== system sampleModel2432_pp_1_2/cfblk239/cfblk15 ==
  cfblk1 : Inport
  Action Port : ActionPort  ActionType=else
  cfblk10 : Delay  ShowEnablePort=on
      settings: InputPortMap=u0,e6
  cfblk3 : DiscreteTransferFcn
  cfblk4 : simulink/Discrete/Transfer Fcn First Order  PoleZ=0.95  ICPrevOutput=0.0  DoSatur=off
      settings: SourceProductName=Simulink
  cfblk5 : DiscreteFir
  cfblk6 : simulink/Discrete/Transfer Fcn First Order  PoleZ=0.95  ICPrevOutput=0.0  DoSatur=off
      settings: SourceProductName=Simulink
  cfblk7 : DiscreteFilter
  cfblk8 : simulink/Discrete/Difference  ICPrevInput=0.0  OutMin=[]  OutMax=[]  OutDataTypeStr=Inherit: Inherit via back propagation  OutDataType=fixdt(1, 16)  OutScaling=2^-10  DoSatur=off
  cfblk9 : DiscreteFilter
  cyemi_{1058..1066} (9 alike) : DataTypeConversion  OutDataTypeStr=double
  cfblk2 : Outport
  cfblk11 : Outport  Port=2
  wires:
  cfblk3/1 -> cfblk2/1
  cfblk4/1 -> cyemi_1062/1, cyemi_1064/1
  cfblk10/1 -> cfblk11/1
  cfblk8/1 -> cyemi_1060/1, cyemi_1063/1
  cyemi_1058/1 -> cfblk10/1
  cfblk6/1 -> cyemi_1058/1
  cyemi_1059/1 -> cfblk10/2
  cfblk7/1 -> cyemi_1059/1
  cyemi_1060/1 -> cfblk3/1
  cyemi_1061/1 -> cfblk4/1
  cfblk9/1 -> cyemi_1061/1
  cyemi_1062/1 -> cfblk5/1
  cyemi_1063/1 -> cfblk6/1
  cyemi_1064/1 -> cfblk7/1
  cyemi_1065/1 -> cfblk8/1
  cfblk5/1 -> cyemi_1065/1
  cyemi_1066/1 -> cfblk9/1
  cfblk1/1 -> cyemi_1066/1

== system sampleModel2432_pp_1_2/cfblk242/cfblk18 ==
  cfblk1 : Inport
  Action Port : ActionPort  ActionType=then
  cfblk12 : Delay
  cfblk3 : DiscreteZeroPole  Poles=[0 0.5]  Gain=1  SampleTime=-1
  cfblk6 : simulink/Discrete/Difference  ICPrevInput=0.0  OutMin=[]  OutMax=[]  OutDataTypeStr=Inherit: Inherit via back propagation  OutDataType=fixdt(1, 16)  OutScaling=2^-10  DoSatur=off
  cfblk8 : DiscreteIntegrator  SampleTime=-1  ICPrevOutput=DiscIntNeverNeededParam  ICPrevScaledInput=DiscIntNeverNeededParam
  cyemi_{1111..1117} (7 alike) : DataTypeConversion  OutDataTypeStr=double
  cfblk2 : Outport
  cfblk9 : Outport  Port=2
  cfblk10 : Outport  Port=3
  cfblk11 : Outport  Port=4
  wires:
  cfblk8/1 -> cfblk2/1
  cfblk1/1 -> cyemi_1115/1, cyemi_1117/1
  cyemi_1111/1 -> cfblk12/1
  cyemi_1112/1 -> cfblk3/1
  cfblk12/1 -> cyemi_1112/1
  cfblk3/1 -> cyemi_1114/1
  cyemi_1115/1 -> cfblk6/1
  cfblk6/1 -> cyemi_1116/1
  cyemi_1117/1 -> cfblk8/1
  cyemi_1113/1 -> cfblk9/1, cfblk11/1, cfblk10/1
  cyemi_1116/1 -> cyemi_1113/1
  cyemi_1114/1 -> cyemi_1111/1

== system sampleModel2432_pp_1_2/cfblk242/cfblk19 ==
  cfblk1 : Inport
  cfblk10 : Inport  Port=2
  Action Port : ActionPort  ActionType=else
  cfblk11 : Delay
  cfblk3 : DiscreteIntegrator  SampleTime=-1  ICPrevOutput=DiscIntNeverNeededParam  ICPrevScaledInput=DiscIntNeverNeededParam
  cfblk4 : simulink/Discrete/Transfer Fcn First Order  PoleZ=0.95  ICPrevOutput=0.0  DoSatur=off
      settings: SourceProductName=Simulink
  cfblk5 : DiscreteStateSpace  SampleTime=-1
  cfblk6 : UnitDelay  SampleTime=-1
  cfblk7 : UnitDelay  SampleTime=-1
  cfblk8 : simulink/Discrete/Transfer Fcn Lead or Lag  PoleZ=0.95  ZeroZ=0.75  ICPrevOutput=0.0  ICPrevInput=0.0  DoSatur=off
      settings: SourceProductName=Simulink  SourceProductBaseCode=SL
  cfblk9 : Delay
  cyemi_{1120..1127} (8 alike) : DataTypeConversion  OutDataTypeStr=double
  cfblk2 : Outport
  wires:
  cfblk5/1 -> cfblk2/1
  cyemi_1120/1 -> cfblk11/1
  cfblk9/1 -> cyemi_1120/1
  cyemi_1121/1 -> cfblk3/1
  cfblk11/1 -> cyemi_1121/1
  cyemi_1122/1 -> cfblk4/1
  cfblk1/1 -> cyemi_1122/1
  cyemi_1123/1 -> cfblk5/1
  cfblk4/1 -> cyemi_1123/1
  cyemi_1124/1 -> cfblk6/1
  cfblk3/1 -> cyemi_1124/1
  cyemi_1125/1 -> cfblk7/1
  cfblk6/1 -> cyemi_1125/1
  cyemi_1126/1 -> cfblk8/1
  cfblk7/1 -> cyemi_1126/1
  cyemi_1127/1 -> cfblk9/1
  cfblk8/1 -> cyemi_1127/1

== system sampleModel2432_pp_1_2/cfblk242/cfblk20 ==
  cfblk1 : Inport
  cfblk13 : Inport  Port=2
  Action Port : ActionPort  ActionType=then
  cfblk11 : simulink/Continuous/PID Controller (2DOF)  Controller=PID  TimeDomain=Discrete-time  SampleTime=-1  IntegratorMethod=Forward Euler  FilterMethod=Forward Euler  Form=Parallel  UseFilter=on  ControllerParametersSource=internal  P=1  I=1  D=0  N=100  b=1  c=1  InitialConditionSource=internal  InitialConditionForIntegrator=0  InitialConditionForFilter=0  ExternalReset=none  LimitOutput=off  UpperSaturationLimit=inf  LowerSaturationLimit=-inf  LinearizeAsGain=off  AntiWindupMode=none  Kb=1  TrackingMode=off  Kt=1  PParamMin=[]  PParamMax=[]  IParamMin=[]  IParamMax=[]  DParamMin=[]  DParamMax=[]  NParamMin=[]  NParamMax=[]  bParamMin=[]  bParamMax=[]  cParamMin=[]  cParamMax=[]  KbParamMin=[]  KbParamMax=[]  KtParamMin=[]  KtParamMax=[]  POutMin=[]  POutMax=[]  IOutMin=[]  IOutMax=[]  DOutMin=[]  DOutMax=[]  NOutMin=[]  NOutMax=[]  bOutMin=[]  bOutMax=[]  cOutMin=[]  cOutMax=[]  KbOutMin=[]  KbOutMax=[]  KtOutMin=[]  KtOutMax=[]  IntegratorOutMin=[]  IntegratorOutMax=[]  FilterOutMin=[]  FilterOutMax=[]  SumOutMin=[]  SumOutMax=[]  Sum1OutMin=[]  Sum1OutMax=[]  Sum2OutMin=[]  Sum2OutMax=[]  Sum3OutMin=[]  Sum3OutMax=[]  SumI1OutMin=[]  SumI1OutMax=[]  SumI2OutMin=[]  SumI2OutMax=[]  SumI3OutMin=[]  SumI3OutMax=[]  SumDOutMin=[]  SumDOutMax=[]  SaturationOutMin=[]  SaturationOutMax=[]  IntegratorContinuousStateAttributes=''  IntegratorStateMustResolveToSignalObject=off  IntegratorRTWStateStorageClass=Auto  FilterContinuousStateAttributes=''  FilterStateMustResolveToSignalObject=off  FilterRTWStateStorageClass=Auto  DifferentiatorICPrevScaledInput=0  DifferentiatorOutMin=[]  DifferentiatorOutMax=[]  FilterDiffOutCoefMin=[]  FilterDiffOutCoefMax=[]  SumDenOutMin=[]  SumDenOutMax=[]  SumNumOutMin=[]  SumNumOutMax=[]  ReciprocalOutMin=[]  ReciprocalOutMax=[]  DivideOutMin=[]  DivideOutMax=[]  TunerSelectOption=Transfer Function Based (PID Tuner App)
  cfblk12 : simulink/Discrete/Tapped Delay  vinit=0.0  samptime=-1  NumDelays=1  DelayOrder=Oldest  includeCurrent=off
  cfblk15 : Delay
  cfblk16 : Delay
  cfblk3 : simulink/Discrete/Difference  ICPrevInput=0.0  OutMin=[]  OutMax=[]  OutDataTypeStr=Inherit: Inherit via back propagation  OutDataType=fixdt(1, 16)  OutScaling=2^-10  DoSatur=off
  cfblk5 : simulink/Continuous/PID Controller  Controller=PID  TimeDomain=Discrete-time  SampleTime=-1  IntegratorMethod=Forward Euler  FilterMethod=Forward Euler  Form=Parallel  UseFilter=on  ControllerParametersSource=internal  P=1  I=1  D=0  N=100  InitialConditionSource=internal  InitialConditionForIntegrator=0  InitialConditionForFilter=0  ExternalReset=none  LimitOutput=off  UpperSaturationLimit=inf  LowerSaturationLimit=-inf  LinearizeAsGain=off  AntiWindupMode=none  Kb=1  TrackingMode=off  Kt=1  PParamMin=[]  PParamMax=[]  IParamMin=[]  IParamMax=[]  DParamMin=[]  DParamMax=[]  NParamMin=[]  NParamMax=[]  KbParamMin=[]  KbParamMax=[]  KtParamMin=[]  KtParamMax=[]  POutMin=[]  POutMax=[]  IOutMin=[]  IOutMax=[]  DOutMin=[]  DOutMax=[]  NOutMin=[]  NOutMax=[]  KbOutMin=[]  KbOutMax=[]  KtOutMin=[]  KtOutMax=[]  IntegratorOutMin=[]  IntegratorOutMax=[]  FilterOutMin=[]  FilterOutMax=[]  SumOutMin=[]  SumOutMax=[]  SumI1OutMin=[]  SumI1OutMax=[]  SumI2OutMin=[]  SumI2OutMax=[]  SumI3OutMin=[]  SumI3OutMax=[]  SumDOutMin=[]  SumDOutMax=[]  SaturationOutMin=[]  SaturationOutMax=[]  IntegratorContinuousStateAttributes=''  IntegratorStateMustResolveToSignalObject=off  IntegratorRTWStateStorageClass=Auto  FilterContinuousStateAttributes=''  FilterStateMustResolveToSignalObject=off  FilterRTWStateStorageClass=Auto  DifferentiatorICPrevScaledInput=0  DifferentiatorOutMin=[]  DifferentiatorOutMax=[]  FilterDiffOutCoefMin=[]  FilterDiffOutCoefMax=[]  SumDenOutMin=[]  SumDenOutMax=[]  SumNumOutMin=[]  SumNumOutMax=[]  ReciprocalOutMin=[]  ReciprocalOutMax=[]  DivideOutMin=[]  DivideOutMax=[]  TunerSelectOption=Transfer Function Based (PID Tuner App)
  cfblk6 : simulink/Discrete/Difference  ICPrevInput=0.0  OutMin=[]  OutMax=[]  OutDataTypeStr=Inherit: Inherit via back propagation  OutDataType=fixdt(1, 16)  OutScaling=2^-10  DoSatur=off
  cfblk7 : simulink/Discrete/Tapped Delay  vinit=0.0  samptime=-1  NumDelays=1  DelayOrder=Oldest  includeCurrent=off
  cfblk9 : simulink/Discrete/Tapped Delay  vinit=0.0  samptime=-1  NumDelays=1  DelayOrder=Oldest  includeCurrent=off
  cyemi_{1130..1142} (13 alike) : DataTypeConversion  OutDataTypeStr=double
  cfblk2 : Outport
  cfblk14 : Outport  Port=2
  wires:
  cfblk3/1 -> cyemi_1139/1, cyemi_1141/1
  cfblk5/1 -> cfblk2/1
  cfblk11/1 -> cfblk14/1
  cfblk9/1 -> cyemi_1130/1
  cyemi_1131/1 -> cfblk11/1
  cfblk12/1 -> cyemi_1131/1
  cyemi_1132/1 -> cfblk11/2
  cfblk7/1 -> cyemi_1132/1
  cyemi_1133/1 -> cfblk12/1
  cfblk6/1 -> cyemi_1133/1
  cyemi_1134/1 -> cfblk15/1
  cyemi_1135/1 -> cfblk16/1
  cyemi_1136/1 -> cfblk3/1
  cfblk15/1 -> cyemi_1136/1
  cfblk16/1 -> cyemi_1137/1
  cyemi_1138/1 -> cfblk5/1
  cfblk1/1 -> cyemi_1138/1
  cyemi_1139/1 -> cfblk6/1
  cyemi_1140/1 -> cfblk7/1
  cfblk13/1 -> cyemi_1140/1
  cyemi_1142/1 -> cfblk9/1
  cyemi_1130/1 -> cyemi_1135/1
  cyemi_1141/1 -> cyemi_1134/1
  cyemi_1137/1 -> cyemi_1142/1

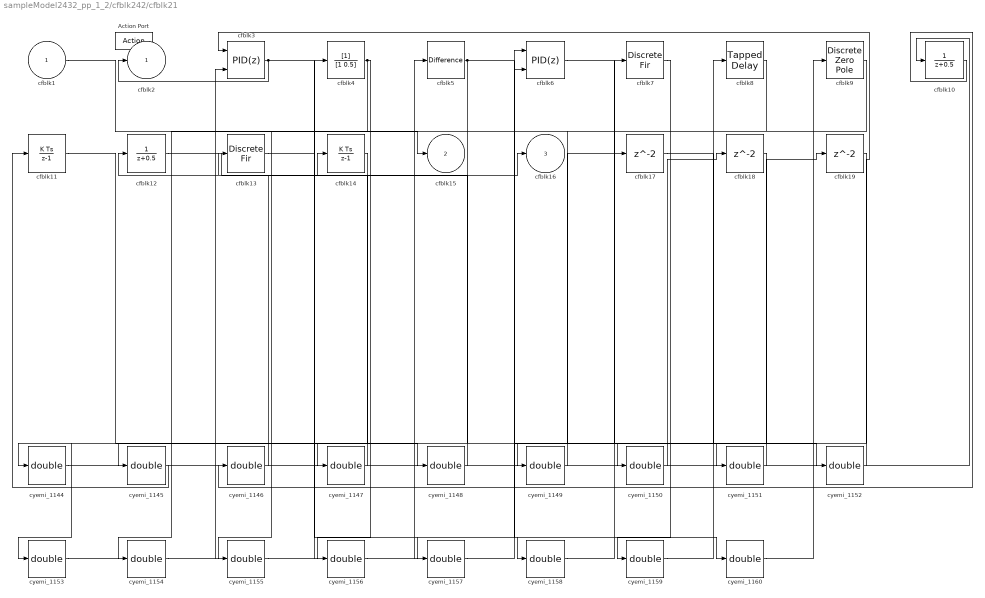
== system sampleModel2432_pp_1_2/cfblk242/cfblk21 ==
  cfblk1 : Inport
  Action Port : ActionPort  ActionType=else
  cfblk10 : DiscreteTransferFcn
  cfblk11 : DiscreteIntegrator  SampleTime=-1  ICPrevOutput=DiscIntNeverNeededParam  ICPrevScaledInput=DiscIntNeverNeededParam
  cfblk12 : DiscreteTransferFcn
  cfblk13 : DiscreteFir
  cfblk14 : DiscreteIntegrator  SampleTime=-1  ICPrevOutput=DiscIntNeverNeededParam  ICPrevScaledInput=DiscIntNeverNeededParam
  cfblk17 : Delay
  cfblk18 : Delay
  cfblk19 : Delay
  cfblk3 : simulink/Continuous/PID Controller (2DOF)  Controller=PID  TimeDomain=Discrete-time  SampleTime=-1  IntegratorMethod=Forward Euler  FilterMethod=Forward Euler  Form=Parallel  UseFilter=on  ControllerParametersSource=internal  P=1  I=1  D=0  N=100  b=1  c=1  InitialConditionSource=internal  InitialConditionForIntegrator=0  InitialConditionForFilter=0  ExternalReset=none  LimitOutput=off  UpperSaturationLimit=inf  LowerSaturationLimit=-inf  LinearizeAsGain=off  AntiWindupMode=none  Kb=1  TrackingMode=off  Kt=1  PParamMin=[]  PParamMax=[]  IParamMin=[]  IParamMax=[]  DParamMin=[]  DParamMax=[]  NParamMin=[]  NParamMax=[]  bParamMin=[]  bParamMax=[]  cParamMin=[]  cParamMax=[]  KbParamMin=[]  KbParamMax=[]  KtParamMin=[]  KtParamMax=[]  POutMin=[]  POutMax=[]  IOutMin=[]  IOutMax=[]  DOutMin=[]  DOutMax=[]  NOutMin=[]  NOutMax=[]  bOutMin=[]  bOutMax=[]  cOutMin=[]  cOutMax=[]  KbOutMin=[]  KbOutMax=[]  KtOutMin=[]  KtOutMax=[]  IntegratorOutMin=[]  IntegratorOutMax=[]  FilterOutMin=[]  FilterOutMax=[]  SumOutMin=[]  SumOutMax=[]  Sum1OutMin=[]  Sum1OutMax=[]  Sum2OutMin=[]  Sum2OutMax=[]  Sum3OutMin=[]  Sum3OutMax=[]  SumI1OutMin=[]  SumI1OutMax=[]  SumI2OutMin=[]  SumI2OutMax=[]  SumI3OutMin=[]  SumI3OutMax=[]  SumDOutMin=[]  SumDOutMax=[]  SaturationOutMin=[]  SaturationOutMax=[]  IntegratorContinuousStateAttributes=''  IntegratorStateMustResolveToSignalObject=off  IntegratorRTWStateStorageClass=Auto  FilterContinuousStateAttributes=''  FilterStateMustResolveToSignalObject=off  FilterRTWStateStorageClass=Auto  DifferentiatorICPrevScaledInput=0  DifferentiatorOutMin=[]  DifferentiatorOutMax=[]  FilterDiffOutCoefMin=[]  FilterDiffOutCoefMax=[]  SumDenOutMin=[]  SumDenOutMax=[]  SumNumOutMin=[]  SumNumOutMax=[]  ReciprocalOutMin=[]  ReciprocalOutMax=[]  DivideOutMin=[]  DivideOutMax=[]  TunerSelectOption=Transfer Function Based (PID Tuner App)
  cfblk4 : DiscreteFilter
  cfblk5 : simulink/Discrete/Difference  ICPrevInput=0.0  OutMin=[]  OutMax=[]  OutDataTypeStr=Inherit: Inherit via back propagation  OutDataType=fixdt(1, 16)  OutScaling=2^-10  DoSatur=off
  cfblk6 : simulink/Continuous/PID Controller (2DOF)  Controller=PID  TimeDomain=Discrete-time  SampleTime=-1  IntegratorMethod=Forward Euler  FilterMethod=Forward Euler  Form=Parallel  UseFilter=on  ControllerParametersSource=internal  P=1  I=1  D=0  N=100  b=1  c=1  InitialConditionSource=internal  InitialConditionForIntegrator=0  InitialConditionForFilter=0  ExternalReset=none  LimitOutput=off  UpperSaturationLimit=inf  LowerSaturationLimit=-inf  LinearizeAsGain=off  AntiWindupMode=none  Kb=1  TrackingMode=off  Kt=1  PParamMin=[]  PParamMax=[]  IParamMin=[]  IParamMax=[]  DParamMin=[]  DParamMax=[]  NParamMin=[]  NParamMax=[]  bParamMin=[]  bParamMax=[]  cParamMin=[]  cParamMax=[]  KbParamMin=[]  KbParamMax=[]  KtParamMin=[]  KtParamMax=[]  POutMin=[]  POutMax=[]  IOutMin=[]  IOutMax=[]  DOutMin=[]  DOutMax=[]  NOutMin=[]  NOutMax=[]  bOutMin=[]  bOutMax=[]  cOutMin=[]  cOutMax=[]  KbOutMin=[]  KbOutMax=[]  KtOutMin=[]  KtOutMax=[]  IntegratorOutMin=[]  IntegratorOutMax=[]  FilterOutMin=[]  FilterOutMax=[]  SumOutMin=[]  SumOutMax=[]  Sum1OutMin=[]  Sum1OutMax=[]  Sum2OutMin=[]  Sum2OutMax=[]  Sum3OutMin=[]  Sum3OutMax=[]  SumI1OutMin=[]  SumI1OutMax=[]  SumI2OutMin=[]  SumI2OutMax=[]  SumI3OutMin=[]  SumI3OutMax=[]  SumDOutMin=[]  SumDOutMax=[]  SaturationOutMin=[]  SaturationOutMax=[]  IntegratorContinuousStateAttributes=''  IntegratorStateMustResolveToSignalObject=off  IntegratorRTWStateStorageClass=Auto  FilterContinuousStateAttributes=''  FilterStateMustResolveToSignalObject=off  FilterRTWStateStorageClass=Auto  DifferentiatorICPrevScaledInput=0  DifferentiatorOutMin=[]  DifferentiatorOutMax=[]  FilterDiffOutCoefMin=[]  FilterDiffOutCoefMax=[]  SumDenOutMin=[]  SumDenOutMax=[]  SumNumOutMin=[]  SumNumOutMax=[]  ReciprocalOutMin=[]  ReciprocalOutMax=[]  DivideOutMin=[]  DivideOutMax=[]  TunerSelectOption=Transfer Function Based (PID Tuner App)
  cfblk7 : DiscreteFir
  cfblk8 : simulink/Discrete/Tapped Delay  vinit=0.0  samptime=-1  NumDelays=1  DelayOrder=Oldest  includeCurrent=off
  cfblk9 : DiscreteZeroPole  Poles=[0 0.5]  Gain=1  SampleTime=-1
  cyemi_{1144..1160} (17 alike) : DataTypeConversion  OutDataTypeStr=double
  cfblk2 : Outport
  cfblk15 : Outport  Port=2
  cfblk16 : Outport  Port=3
  wires:
  cfblk3/1 -> cfblk2/1, cyemi_1158/1
  cfblk4/1 -> cyemi_1145/1, cyemi_1156/1
  cfblk12/1 -> cfblk16/1
  cfblk5/1 -> cyemi_1144/1, cyemi_1150/1, cyemi_1160/1
  cfblk1/1 -> cfblk15/1
  cyemi_1144/1 -> cfblk10/1
  cyemi_1145/1 -> cfblk11/1
  cyemi_1146/1 -> cfblk12/1
  cfblk10/1 -> cyemi_1146/1
  cyemi_1147/1 -> cfblk13/1
  cfblk14/1 -> cyemi_1147/1
  cyemi_1148/1 -> cfblk14/1
  cfblk11/1 -> cyemi_1148/1
  cyemi_1149/1 -> cfblk17/1
  cfblk9/1 -> cyemi_1149/1
  cyemi_1150/1 -> cfblk18/1
  cyemi_1151/1 -> cfblk19/1
  cfblk6/1 -> cyemi_1151/1
  cyemi_1152/1 -> cfblk3/1
  cfblk17/1 -> cyemi_1152/1
  cyemi_1153/1 -> cfblk3/2
  cfblk18/1 -> cyemi_1153/1
  cyemi_1154/1 -> cfblk4/1
  cfblk19/1 -> cyemi_1154/1
  cyemi_1155/1 -> cfblk5/1
  cfblk8/1 -> cyemi_1155/1
  cyemi_1156/1 -> cfblk6/1
  cyemi_1157/1 -> cfblk6/2
  cfblk13/1 -> cyemi_1157/1
  cyemi_1158/1 -> cfblk7/1
  cyemi_1159/1 -> cfblk8/1
  cfblk7/1 -> cyemi_1159/1
  cyemi_1160/1 -> cfblk9/1

== system sampleModel2432_pp_1_2/cfblk243/cfblk13 ==
  cfblk1 : Inport
  cfblk10 : Inport  Port=2
  Action Port : ActionPort
  cfblk11 : Delay
  cfblk3 : simulink/Continuous/PID Controller  Controller=PID  TimeDomain=Discrete-time  SampleTime=-1  IntegratorMethod=Forward Euler  FilterMethod=Forward Euler  Form=Parallel  UseFilter=on  ControllerParametersSource=internal  P=1  I=1  D=0  N=100  InitialConditionSource=internal  InitialConditionForIntegrator=0  InitialConditionForFilter=0  ExternalReset=none  LimitOutput=off  UpperSaturationLimit=inf  LowerSaturationLimit=-inf  LinearizeAsGain=off  AntiWindupMode=none  Kb=1  TrackingMode=off  Kt=1  PParamMin=[]  PParamMax=[]  IParamMin=[]  IParamMax=[]  DParamMin=[]  DParamMax=[]  NParamMin=[]  NParamMax=[]  KbParamMin=[]  KbParamMax=[]  KtParamMin=[]  KtParamMax=[]  POutMin=[]  POutMax=[]  IOutMin=[]  IOutMax=[]  DOutMin=[]  DOutMax=[]  NOutMin=[]  NOutMax=[]  KbOutMin=[]  KbOutMax=[]  KtOutMin=[]  KtOutMax=[]  IntegratorOutMin=[]  IntegratorOutMax=[]  FilterOutMin=[]  FilterOutMax=[]  SumOutMin=[]  SumOutMax=[]  SumI1OutMin=[]  SumI1OutMax=[]  SumI2OutMin=[]  SumI2OutMax=[]  SumI3OutMin=[]  SumI3OutMax=[]  SumDOutMin=[]  SumDOutMax=[]  SaturationOutMin=[]  SaturationOutMax=[]  IntegratorContinuousStateAttributes=''  IntegratorStateMustResolveToSignalObject=off  IntegratorRTWStateStorageClass=Auto  FilterContinuousStateAttributes=''  FilterStateMustResolveToSignalObject=off  FilterRTWStateStorageClass=Auto  DifferentiatorICPrevScaledInput=0  DifferentiatorOutMin=[]  DifferentiatorOutMax=[]  FilterDiffOutCoefMin=[]  FilterDiffOutCoefMax=[]  SumDenOutMin=[]  SumDenOutMax=[]  SumNumOutMin=[]  SumNumOutMax=[]  ReciprocalOutMin=[]  ReciprocalOutMax=[]  DivideOutMin=[]  DivideOutMax=[]  TunerSelectOption=Transfer Function Based (PID Tuner App)
  cfblk4 : simulink/Discrete/Transfer Fcn First Order  PoleZ=0.95  ICPrevOutput=0.0  DoSatur=off
      settings: SourceProductName=Simulink
  cfblk5 : DiscreteStateSpace  SampleTime=-1
  cfblk7 : simulink/Discrete/Transfer Fcn First Order  PoleZ=0.95  ICPrevOutput=0.0  DoSatur=off
      settings: SourceProductName=Simulink
  cyemi_{1181..1188} (8 alike) : DataTypeConversion  OutDataTypeStr=double
  cfblk2 : Outport
  wires:
  cfblk3/1 -> cfblk2/1
  cyemi_1181/1 -> cfblk11/1
  cfblk5/1 -> cyemi_1181/1
  cyemi_1182/1 -> cfblk3/1
  cyemi_1183/1 -> cfblk4/1
  cfblk11/1 -> cyemi_1183/1
  cyemi_1184/1 -> cfblk5/1
  cfblk7/1 -> cyemi_1184/1
  cfblk1/1 -> cyemi_1185/1
  cyemi_1186/1 -> cfblk7/1
  cfblk4/1 -> cyemi_1188/1
  cyemi_1188/1 -> cyemi_1187/1
  cyemi_1187/1 -> cyemi_1186/1
  cyemi_1185/1 -> cyemi_1182/1
